simulink model "ex3_dataflow"  (R2024a)
settings: Solver=VariableStepAuto  StartTime=0.0  StopTime=10.0  RelTol=1e-3
undefined symbols (not defined in the file): designMultirateFIR
libraries: dspmlti4 x4, dspindex x3
settings Model: Creator=erfuu  LastModifiedBy=erfuu
settings OptimizationCC: SimCompilerOptimization=on
settings DebuggingCC: IntegerOverflowMsg=none  IntegerSaturationMsg=none
settings SFSimCC: SimCtrlC=off

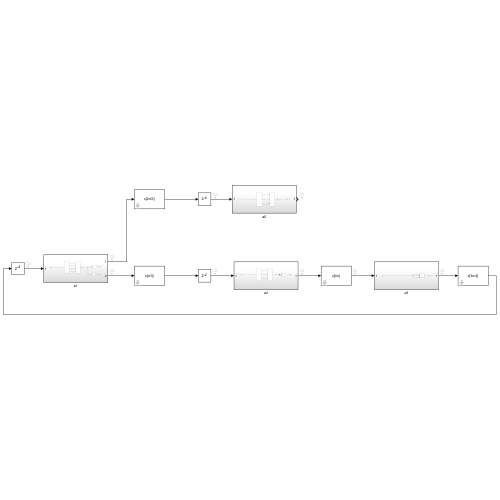
[thumbnail: Simulink's stored preview of the top-level diagram]
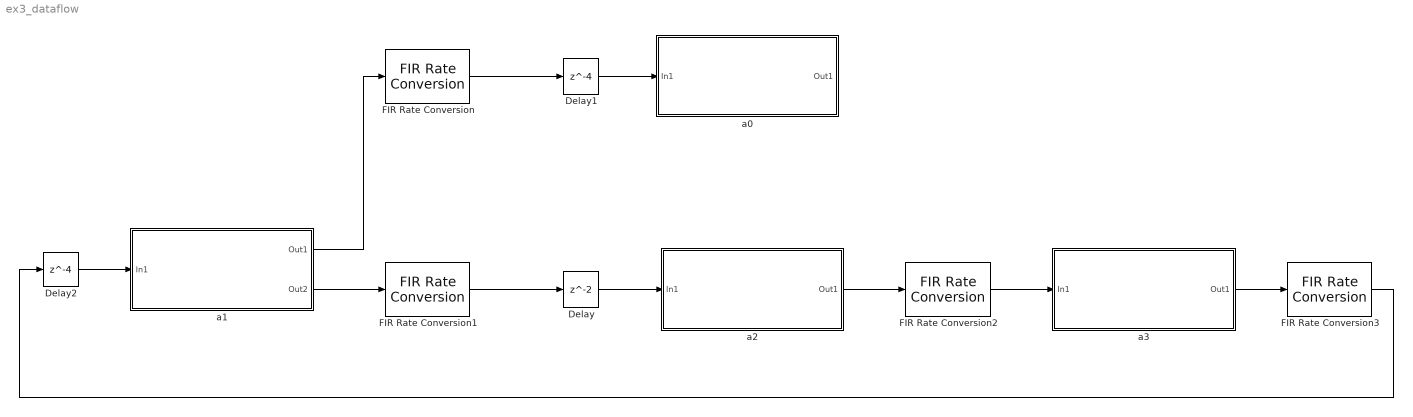
== system ex3_dataflow ==
  Delay : Delay  InitialCondition=1
  Delay1 : Delay  DelayLength=4  InitialCondition=3
  Delay2 : Delay  DelayLength=4  InitialCondition=2
  FIR Rate Conversion : dspmlti4/FIR Rate Conversion  FilterSource=Auto  L=3  h=designMultirateFIR(3,2)  M=2  FilterObject=FRC  rateMode=Enforce single-rate processing  AllowArbitraryInputLength=off  roundingMode=Floor  overflowMode=off  firstCoeffDataTypeStr=Inherit: Same word length as input  firstCoeffMin=[]  firstCoeffMax=[]  firstCoeffLastDataTypeStr=Inherit: Same word length as input  outputDataTypeStr=Inherit: Same as accumulator  outputMin=[]  outputMax=[]  outputLastDataTypeStr=Inherit: Same as accumulator
  FIR Rate Conversion1 : dspmlti4/FIR Rate Conversion  FilterSource=Auto  L=3  h=designMultirateFIR(3,2)  M=1  FilterObject=FRC  rateMode=Enforce single-rate processing  AllowArbitraryInputLength=off  roundingMode=Floor  overflowMode=off  firstCoeffDataTypeStr=Inherit: Same word length as input  firstCoeffMin=[]  firstCoeffMax=[]  firstCoeffLastDataTypeStr=Inherit: Same word length as input  outputDataTypeStr=Inherit: Same as accumulator  outputMin=[]  outputMax=[]  outputLastDataTypeStr=Inherit: Same as accumulator
  FIR Rate Conversion2 : dspmlti4/FIR Rate Conversion  FilterSource=Auto  L=1  h=designMultirateFIR(3,2)  M=4  FilterObject=FRC  rateMode=Enforce single-rate processing  AllowArbitraryInputLength=off  roundingMode=Floor  overflowMode=off  firstCoeffDataTypeStr=Inherit: Same word length as input  firstCoeffMin=[]  firstCoeffMax=[]  firstCoeffLastDataTypeStr=Inherit: Same word length as input  outputDataTypeStr=Inherit: Same as accumulator  outputMin=[]  outputMax=[]  outputLastDataTypeStr=Inherit: Same as accumulator
  FIR Rate Conversion3 : dspmlti4/FIR Rate Conversion  FilterSource=Auto  L=4  h=designMultirateFIR(3,2)  M=3  FilterObject=FRC  rateMode=Enforce single-rate processing  AllowArbitraryInputLength=off  roundingMode=Floor  overflowMode=off  firstCoeffDataTypeStr=Inherit: Same word length as input  firstCoeffMin=[]  firstCoeffMax=[]  firstCoeffLastDataTypeStr=Inherit: Same word length as input  outputDataTypeStr=Inherit: Same as accumulator  outputMin=[]  outputMax=[]  outputLastDataTypeStr=Inherit: Same as accumulator
  a0 : Subsystem  AutoFrameSizeCalculation=on
  a1 : Subsystem  AutoFrameSizeCalculation=on
  a2 : Subsystem  AutoFrameSizeCalculation=on
  a3 : Subsystem  AutoFrameSizeCalculation=on
  wires:
  a1/1(Out1) -> FIR Rate Conversion/1
  a1/2(Out2) -> FIR Rate Conversion1/1
  a2/1(Out1) -> FIR Rate Conversion2/1
  a3/1(Out1) -> FIR Rate Conversion3/1
  FIR Rate Conversion/1 -> Delay1/1
  Delay1/1 -> a0/1(In1)
  FIR Rate Conversion1/1 -> Delay/1
  Delay/1 -> a2/1(In1)
  FIR Rate Conversion2/1 -> a3/1(In1)
  Delay2/1 -> a1/1(In1)
  FIR Rate Conversion3/1 -> Delay2/1

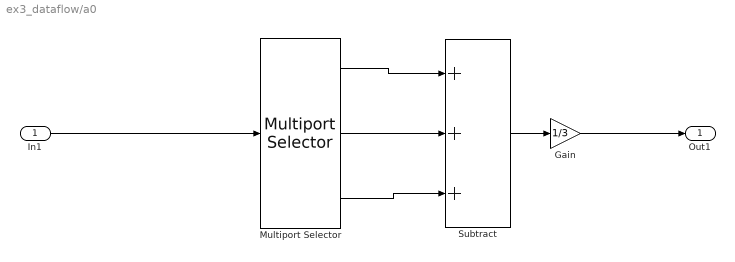
== system ex3_dataflow/a0 ==
  In1 : Inport
  Gain : Gain  Gain=1/3
  Multiport Selector : dspindex/Multiport Selector  rowsOrCols=Rows  idxCellArray={ 1, 2, 3 }  idxErrMode=Clip Index
  Subtract : Sum  Inputs=+++
  Out1 : Outport
  wires:
  Gain/1 -> Out1/1
  Multiport Selector/2 -> Subtract/2
  In1/1 -> Multiport Selector/1
  Subtract/1 -> Gain/1
  Multiport Selector/1 -> Subtract/1
  Multiport Selector/3 -> Subtract/3

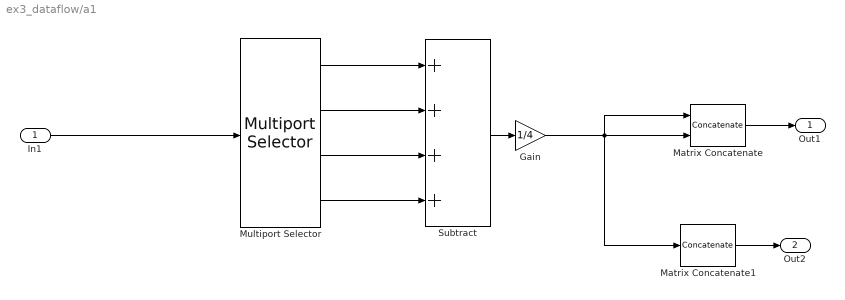
== system ex3_dataflow/a1 ==
  In1 : Inport
  Gain : Gain  Gain=1/4
  Matrix Concatenate : Concatenate  ConcatenateDimension=2
  Matrix Concatenate1 : Concatenate  NumInputs=1  ConcatenateDimension=2
  Multiport Selector : dspindex/Multiport Selector  rowsOrCols=Rows  idxCellArray={ 1, 2, 3, 4 }  idxErrMode=Clip Index
  Subtract : Sum  Inputs=++++
  Out1 : Outport  VectorParamsAs1DForOutWhenUnconnected=off
  Out2 : Outport  Port=2  VectorParamsAs1DForOutWhenUnconnected=off
  wires:
  Gain/1 -> Matrix Concatenate1/1, Matrix Concatenate/2, Matrix Concatenate/1
  Matrix Concatenate/1 -> Out1/1
  Multiport Selector/3 -> Subtract/3
  Multiport Selector/4 -> Subtract/4
  Multiport Selector/1 -> Subtract/1
  Multiport Selector/2 -> Subtract/2
  In1/1 -> Multiport Selector/1
  Subtract/1 -> Gain/1
  Matrix Concatenate1/1 -> Out2/1

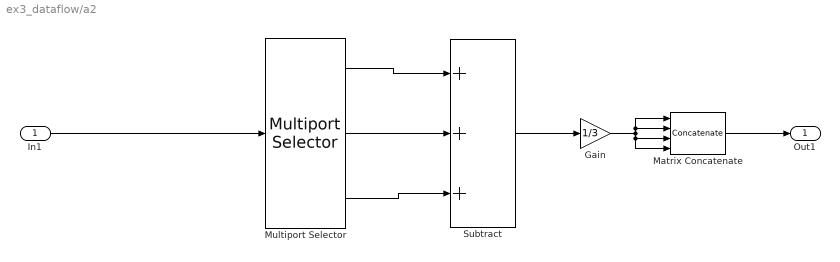
== system ex3_dataflow/a2 ==
  In1 : Inport
  Gain : Gain  Gain=1/3
  Matrix Concatenate : Concatenate  NumInputs=4  ConcatenateDimension=2
  Multiport Selector : dspindex/Multiport Selector  rowsOrCols=Rows  idxCellArray={ 1, 2, 3 }  idxErrMode=Clip Index
  Subtract : Sum  Inputs=+++
  Out1 : Outport  VectorParamsAs1DForOutWhenUnconnected=off
  wires:
  Gain/1 -> Matrix Concatenate/4, Matrix Concatenate/3, Matrix Concatenate/2, Matrix Concatenate/1
  Matrix Concatenate/1 -> Out1/1
  Multiport Selector/2 -> Subtract/2
  In1/1 -> Multiport Selector/1
  Subtract/1 -> Gain/1
  Multiport Selector/1 -> Subtract/1
  Multiport Selector/3 -> Subtract/3

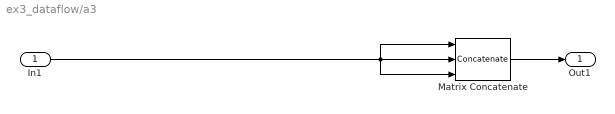
== system ex3_dataflow/a3 ==
  In1 : Inport
  Matrix Concatenate : Concatenate  NumInputs=3  ConcatenateDimension=2
  Out1 : Outport  VectorParamsAs1DForOutWhenUnconnected=off
  wires:
  In1/1 -> Matrix Concatenate/3, Matrix Concatenate/2, Matrix Concatenate/1
  Matrix Concatenate/1 -> Out1/1
